simulink model "sb_cross_mult_core"  (R2012b)
settings: Solver=ode45  StartTime=0.0  StopTime=10.0  RelTol=1e-3
libraries: xbsIndex_r4 x485, casper_library_misc x72
(part 1 of 5)
settings Model: Creator=jack  LastModifiedBy=jack

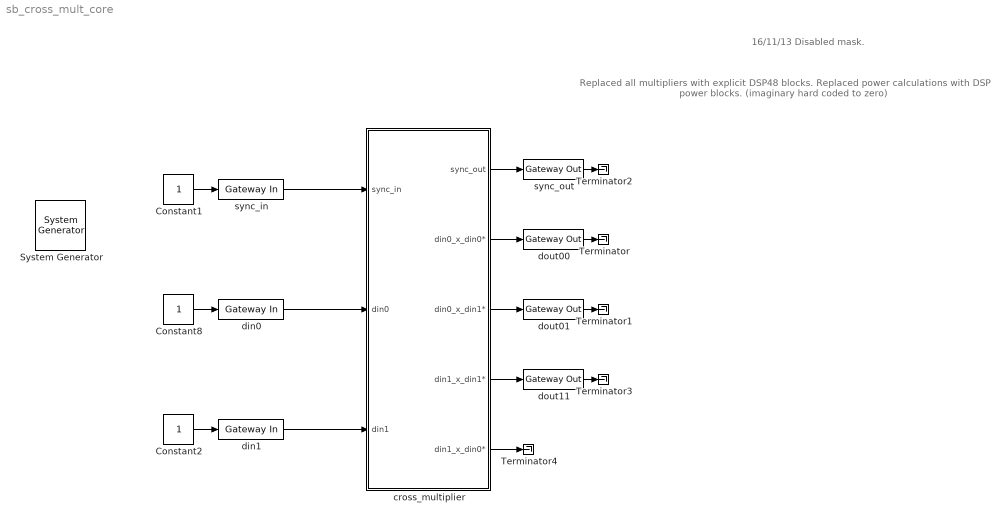
== system sb_cross_mult_core ==
  note: Replaced all multipliers with explicit DSP48 blocks.
      | Replaced power calculations with DSP power blocks. (imaginary hard coded to zero)
  note: 16/11/13
      | Disabled mask.
  " System Generator" : xbsIndex_r4/ System Generator  Tag=genX  xilinxfamily=virtex6  part=xc6vsx475t  speed=-1  package=ff1759  synthesis_tool=XST  clock_wrapper=Clock Enables  directory=./sb_cross_mult_core  proj_type=Project Navigator  Synth_file=XST Defaults  Impl_file=ISE Defaults  testbench=off  simulink_period=1  sysclk_period=3.2  dcm_input_clock_period=10  incr_netlist=off  trim_vbits=Everywhere in SubSystem  dbl_ovrd=According to Block Masks  core_generation=According to Block Masks  run_coregen=off  deprecated_control=off  eval_field=0  block_type=sysgen
  Constant1 : Constant
  Constant2 : Constant
  Constant8 : Constant
  Terminator{,1..4} (5 alike) : Terminator
  cross_multiplier : Subsystem  mask(cross_multiplier){streams=2, aggregation=8, bit_width_in=4, binary_point_in=3, bit_width_out=9, binary_point_out=6, mult_latency=3, add_latency=1, overflow=Wrap, quantisation=Truncate, conv_latency=0}
      mask prompts: streams "Number input streams"; aggregation "Aggregation per stream"; bit_width_in "Bit width in"; binary_point_in "Binary point in"; bit_width_out "Bit width out"; binary_point_out "Binary point out"; mult_latency "Multiplier latency"; add_latency "Adder latency"; overflow "Overflow behaviour"; quantisation "Quantisation behaviour"; conv_latency "Bit width conversion latency"
      mask help: Cross multiplies aggregated complex input streams.
      mask init:
      | % cross_multiplier_init(gcb, ...
      | %     'streams', streams, ...
      | %     'aggregation', aggregation, ...
      | %     'bit_width_in', bit_width_in, ...
      | %     'binary_point_in', binary_point_in, ...
      | %     'bit_width_out', bit_width_out, ...
      | %     'binary_point_out', binary_point_out, ...
      | %     'mult_latency', mult_latency, ...
      | %     'add_latency', add_latency, ...
      | %     'overflow', overflow, ...
      | %     'quantisation', quantisation, ...
      | %     'conv_latency', conv_latency);
      mask TypeOptions overflow: Wrap | Saturate | Error
      mask TypeOptions quantisation: Truncate | Round  (unbiased: +/- Inf) | Round  (unbiased: even values)
  din0 : xbsIndex_r4/Gateway In  gui_display_data_type=Fixed-point  arith_type=Unsigned  n_bits=8*8  bin_pt=0  preci_type=Single  exp_width=8  frac_width=24  quantization="Round  (unbiased: +/- Inf)"  overflow=Saturate  period=1  dbl_ovrd=off  timing_constraint=None  locs_specified=off  LOCs={}  UseAsADC=off  ADCChannel='1'  inherit_from_input=off  hdl_port=on  block_type=gatewayin
  din1 : xbsIndex_r4/Gateway In  gui_display_data_type=Fixed-point  arith_type=Unsigned  n_bits=8*8  bin_pt=0  preci_type=Single  exp_width=8  frac_width=24  quantization="Round  (unbiased: +/- Inf)"  overflow=Saturate  period=1  dbl_ovrd=off  timing_constraint=None  locs_specified=off  LOCs={}  UseAsADC=off  ADCChannel='1'  inherit_from_input=off  hdl_port=on  block_type=gatewayin
  dout00 : xbsIndex_r4/Gateway Out  inherit_from_input=off  hdl_port=on  timing_constraint=None  locs_specified=off  LOCs={}  UseAsDAC=off  DACChannel='1'  block_type=gatewayout
  dout01 : xbsIndex_r4/Gateway Out  inherit_from_input=off  hdl_port=on  timing_constraint=None  locs_specified=off  LOCs={}  UseAsDAC=off  DACChannel='1'  block_type=gatewayout
  dout11 : xbsIndex_r4/Gateway Out  inherit_from_input=off  hdl_port=on  timing_constraint=None  locs_specified=off  LOCs={}  UseAsDAC=off  DACChannel='1'  block_type=gatewayout
  sync_in : xbsIndex_r4/Gateway In  gui_display_data_type=Boolean  arith_type=Boolean  n_bits=16  bin_pt=14  preci_type=Single  exp_width=8  frac_width=24  quantization="Round  (unbiased: +/- Inf)"  overflow=Saturate  period=1  dbl_ovrd=off  timing_constraint=None  locs_specified=off  LOCs={}  UseAsADC=off  ADCChannel='1'  inherit_from_input=off  hdl_port=on  block_type=gatewayin
  sync_out : xbsIndex_r4/Gateway Out  inherit_from_input=off  hdl_port=on  timing_constraint=None  locs_specified=off  LOCs={}  UseAsDAC=off  DACChannel='1'  block_type=gatewayout
  wires:
  Constant1/1 -> sync_in/1
  dout00/1 -> Terminator/1
  sync_out/1 -> Terminator2/1
  Constant8/1 -> din0/1
  cross_multiplier/1(sync_out) -> sync_out/1
  cross_multiplier/2(din0_x_din0*) -> dout00/1
  dout01/1 -> Terminator1/1
  cross_multiplier/3(din0_x_din1*) -> dout01/1
  dout11/1 -> Terminator3/1
  cross_multiplier/4(din1_x_din1*) -> dout11/1
  cross_multiplier/5(din1_x_din0*) -> Terminator4/1
  sync_in/1 -> cross_multiplier/1(sync_in)
  din0/1 -> cross_multiplier/2(din0)
  Constant2/1 -> din1/1
  din1/1 -> cross_multiplier/3(din1)

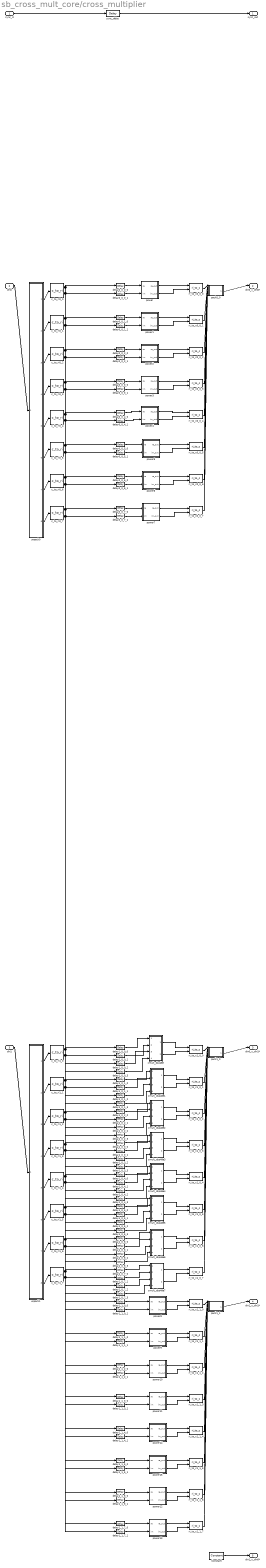
== system sb_cross_mult_core/cross_multiplier ==
  sync_in : Inport
  din0 : Inport  Port=2
  din1 : Inport  Port=3
  Constant : xbsIndex_r4/Constant  const=0  gui_display_data_type=Fixed-point  arith_type=Unsigned  n_bits=2*9*8  bin_pt=0  preci_type=Single  exp_width=8  frac_width=24  explicit_period=on  period=1  equ=P=C  opselect=C  inp2=PCIN>>17  opr=+  inp1=P  carry=CIN  dbl_ovrd=off  block_type=constant
  c_to_ri0_{0..7} (8 alike) : casper_library_misc/c_to_ri  n_bits=bit_width_in  bin_pt=binary_point_in
      settings: AttributesFormatString=4_3 r/i
  c_to_ri1_{0..7} (8 alike) : casper_library_misc/c_to_ri  n_bits=bit_width_in  bin_pt=binary_point_in
      settings: AttributesFormatString=4_3 r/i
  cmult_dsp48e : Subsystem  AncestorBlock=casper_library_multipliers/cmult_dsp48e  mask(cmult_dsp48e){n_bits_a=4, bin_pt_a=3, n_bits_b=4, bin_pt_b=3, conjugated=on, full_precision=on, n_bits_c=37, bin_pt_c=34, quantization=Truncate, overflow=Wrap, cast_latency=0}
      mask prompts: n_bits_a "Bit width 'a'"; bin_pt_a "Binary point 'a'"; n_bits_b "Bit width 'b'"; bin_pt_b "Binary point 'b'"; conjugated "Conjugate"; full_precision "Full precision"; n_bits_c "Bit width out"; bin_pt_c "Binary point out"; cast_latency "Cast Latency"
      mask help:
      | Multiplies two complex numbers using 4 DSP48Es.
      | Conjugation is optional.
      |
      | Re{a} and Im{a} can be up to 25 bits.
      | Re{b} and Im{b} can be up to 18 bits.
      mask init:
      | cmult_dsp48e_init(gcb, ...
      |     'n_bits_a', n_bits_a, ...
      |     'bin_pt_a', bin_pt_a, ...
      |     'n_bits_b', n_bits_b, ...
      |     'bin_pt_b', bin_pt_b, ...
      |     'conjugated', conjugated, ...
      |     'full_precision', full_precision, ...
      |     'n_bits_c', n_bits_c, ...
      |     'bin_pt_c', bin_pt_c, ...
      |     'quantization', quantization, ...
      |     'overflow', overflow, ...
      |     'cast_latency', cast_latency);
      settings: AttributesFormatString=|
      | 4_3 * 4_3 ==> 9_6
      | Latency=4
      mask Callback full_precision:
      | full_precision = get_param(gcb, 'full_precision');
      | 
      | if strcmp(full_precision, 'on'),
      |     not_full_precision = 'off';
      | else
      |     not_full_precision = 'on';
      | end
      | 
      | set_param_state(gcb, 'n_bits_c', not_full_precision);
      | set_param_state(gcb, 'bin_pt_c', not_full_precision);
      | set_param_state(gcb, 'quantization', not_full_precision);
      | set_param_state(gcb, 'overflow', not_full_precision);
      | set_param_state(gcb, 'cast_latency', not_full_precision);
      mask TypeOptions quantization: Truncate | Round  (unbiased: +/- Inf) | Round  (unbiased: Even Values)
      mask TypeOptions overflow: Wrap | Saturate | Flag as error
  cmult_dsp48e1 : Subsystem  AncestorBlock=casper_library_multipliers/cmult_dsp48e  mask(cmult_dsp48e){n_bits_a=4, bin_pt_a=3, n_bits_b=4, bin_pt_b=3, conjugated=on, full_precision=on, n_bits_c=37, bin_pt_c=34, quantization=Truncate, overflow=Wrap, cast_latency=0}
      mask prompts: n_bits_a "Bit width 'a'"; bin_pt_a "Binary point 'a'"; n_bits_b "Bit width 'b'"; bin_pt_b "Binary point 'b'"; conjugated "Conjugate"; full_precision "Full precision"; n_bits_c "Bit width out"; bin_pt_c "Binary point out"; cast_latency "Cast Latency"
      mask help:
      | Multiplies two complex numbers using 4 DSP48Es.
      | Conjugation is optional.
      |
      | Re{a} and Im{a} can be up to 25 bits.
      | Re{b} and Im{b} can be up to 18 bits.
      mask init: same as sb_cross_mult_core/cross_multiplier/cmult_dsp48e
      settings: AttributesFormatString=|
      | 4_3 * 4_3 ==> 9_6
      | Latency=4
      mask Callback full_precision:
      | full_precision = get_param(gcb, 'full_precision');
      | 
      | if strcmp(full_precision, 'on'),
      |     not_full_precision = 'off';
      | else
      |     not_full_precision = 'on';
      | end
      | 
      | set_param_state(gcb, 'n_bits_c', not_full_precision);
      | set_param_state(gcb, 'bin_pt_c', not_full_precision);
      | set_param_state(gcb, 'quantization', not_full_precision);
      | set_param_state(gcb, 'overflow', not_full_precision);
      | set_param_state(gcb, 'cast_latency', not_full_precision);
      mask TypeOptions quantization: Truncate | Round  (unbiased: +/- Inf) | Round  (unbiased: Even Values)
      mask TypeOptions overflow: Wrap | Saturate | Flag as error
  cmult_dsp48e2 : Subsystem  AncestorBlock=casper_library_multipliers/cmult_dsp48e  mask(cmult_dsp48e){n_bits_a=4, bin_pt_a=3, n_bits_b=4, bin_pt_b=3, conjugated=on, full_precision=on, n_bits_c=37, bin_pt_c=34, quantization=Truncate, overflow=Wrap, cast_latency=0}
      mask prompts: n_bits_a "Bit width 'a'"; bin_pt_a "Binary point 'a'"; n_bits_b "Bit width 'b'"; bin_pt_b "Binary point 'b'"; conjugated "Conjugate"; full_precision "Full precision"; n_bits_c "Bit width out"; bin_pt_c "Binary point out"; cast_latency "Cast Latency"
      mask help:
      | Multiplies two complex numbers using 4 DSP48Es.
      | Conjugation is optional.
      |
      | Re{a} and Im{a} can be up to 25 bits.
      | Re{b} and Im{b} can be up to 18 bits.
      mask init: same as sb_cross_mult_core/cross_multiplier/cmult_dsp48e
      settings: AttributesFormatString=|
      | 4_3 * 4_3 ==> 9_6
      | Latency=4
      mask Callback full_precision:
      | full_precision = get_param(gcb, 'full_precision');
      | 
      | if strcmp(full_precision, 'on'),
      |     not_full_precision = 'off';
      | else
      |     not_full_precision = 'on';
      | end
      | 
      | set_param_state(gcb, 'n_bits_c', not_full_precision);
      | set_param_state(gcb, 'bin_pt_c', not_full_precision);
      | set_param_state(gcb, 'quantization', not_full_precision);
      | set_param_state(gcb, 'overflow', not_full_precision);
      | set_param_state(gcb, 'cast_latency', not_full_precision);
      mask TypeOptions quantization: Truncate | Round  (unbiased: +/- Inf) | Round  (unbiased: Even Values)
      mask TypeOptions overflow: Wrap | Saturate | Flag as error
  cmult_dsp48e3 : Subsystem  AncestorBlock=casper_library_multipliers/cmult_dsp48e  mask(cmult_dsp48e){n_bits_a=4, bin_pt_a=3, n_bits_b=4, bin_pt_b=3, conjugated=on, full_precision=on, n_bits_c=37, bin_pt_c=34, quantization=Truncate, overflow=Wrap, cast_latency=0}
      mask prompts: n_bits_a "Bit width 'a'"; bin_pt_a "Binary point 'a'"; n_bits_b "Bit width 'b'"; bin_pt_b "Binary point 'b'"; conjugated "Conjugate"; full_precision "Full precision"; n_bits_c "Bit width out"; bin_pt_c "Binary point out"; cast_latency "Cast Latency"
      mask help:
      | Multiplies two complex numbers using 4 DSP48Es.
      | Conjugation is optional.
      |
      | Re{a} and Im{a} can be up to 25 bits.
      | Re{b} and Im{b} can be up to 18 bits.
      mask init: same as sb_cross_mult_core/cross_multiplier/cmult_dsp48e
      settings: AttributesFormatString=|
      | 4_3 * 4_3 ==> 9_6
      | Latency=4
      mask Callback full_precision:
      | full_precision = get_param(gcb, 'full_precision');
      | 
      | if strcmp(full_precision, 'on'),
      |     not_full_precision = 'off';
      | else
      |     not_full_precision = 'on';
      | end
      | 
      | set_param_state(gcb, 'n_bits_c', not_full_precision);
      | set_param_state(gcb, 'bin_pt_c', not_full_precision);
      | set_param_state(gcb, 'quantization', not_full_precision);
      | set_param_state(gcb, 'overflow', not_full_precision);
      | set_param_state(gcb, 'cast_latency', not_full_precision);
      mask TypeOptions quantization: Truncate | Round  (unbiased: +/- Inf) | Round  (unbiased: Even Values)
      mask TypeOptions overflow: Wrap | Saturate | Flag as error
  cmult_dsp48e4 : Subsystem  AncestorBlock=casper_library_multipliers/cmult_dsp48e  mask(cmult_dsp48e){n_bits_a=4, bin_pt_a=3, n_bits_b=4, bin_pt_b=3, conjugated=on, full_precision=on, n_bits_c=37, bin_pt_c=34, quantization=Truncate, overflow=Wrap, cast_latency=0}
      mask prompts: n_bits_a "Bit width 'a'"; bin_pt_a "Binary point 'a'"; n_bits_b "Bit width 'b'"; bin_pt_b "Binary point 'b'"; conjugated "Conjugate"; full_precision "Full precision"; n_bits_c "Bit width out"; bin_pt_c "Binary point out"; cast_latency "Cast Latency"
      mask help:
      | Multiplies two complex numbers using 4 DSP48Es.
      | Conjugation is optional.
      |
      | Re{a} and Im{a} can be up to 25 bits.
      | Re{b} and Im{b} can be up to 18 bits.
      mask init: same as sb_cross_mult_core/cross_multiplier/cmult_dsp48e
      settings: AttributesFormatString=|
      | 4_3 * 4_3 ==> 9_6
      | Latency=4
      mask Callback full_precision:
      | full_precision = get_param(gcb, 'full_precision');
      | 
      | if strcmp(full_precision, 'on'),
      |     not_full_precision = 'off';
      | else
      |     not_full_precision = 'on';
      | end
      | 
      | set_param_state(gcb, 'n_bits_c', not_full_precision);
      | set_param_state(gcb, 'bin_pt_c', not_full_precision);
      | set_param_state(gcb, 'quantization', not_full_precision);
      | set_param_state(gcb, 'overflow', not_full_precision);
      | set_param_state(gcb, 'cast_latency', not_full_precision);
      mask TypeOptions quantization: Truncate | Round  (unbiased: +/- Inf) | Round  (unbiased: Even Values)
      mask TypeOptions overflow: Wrap | Saturate | Flag as error
  cmult_dsp48e5 : Subsystem  AncestorBlock=casper_library_multipliers/cmult_dsp48e  mask(cmult_dsp48e){n_bits_a=4, bin_pt_a=3, n_bits_b=4, bin_pt_b=3, conjugated=on, full_precision=on, n_bits_c=37, bin_pt_c=34, quantization=Truncate, overflow=Wrap, cast_latency=0}
      mask prompts: n_bits_a "Bit width 'a'"; bin_pt_a "Binary point 'a'"; n_bits_b "Bit width 'b'"; bin_pt_b "Binary point 'b'"; conjugated "Conjugate"; full_precision "Full precision"; n_bits_c "Bit width out"; bin_pt_c "Binary point out"; cast_latency "Cast Latency"
      mask help:
      | Multiplies two complex numbers using 4 DSP48Es.
      | Conjugation is optional.
      |
      | Re{a} and Im{a} can be up to 25 bits.
      | Re{b} and Im{b} can be up to 18 bits.
      mask init: same as sb_cross_mult_core/cross_multiplier/cmult_dsp48e
      settings: AttributesFormatString=|
      | 4_3 * 4_3 ==> 9_6
      | Latency=4
      mask Callback full_precision:
      | full_precision = get_param(gcb, 'full_precision');
      | 
      | if strcmp(full_precision, 'on'),
      |     not_full_precision = 'off';
      | else
      |     not_full_precision = 'on';
      | end
      | 
      | set_param_state(gcb, 'n_bits_c', not_full_precision);
      | set_param_state(gcb, 'bin_pt_c', not_full_precision);
      | set_param_state(gcb, 'quantization', not_full_precision);
      | set_param_state(gcb, 'overflow', not_full_precision);
      | set_param_state(gcb, 'cast_latency', not_full_precision);
      mask TypeOptions quantization: Truncate | Round  (unbiased: +/- Inf) | Round  (unbiased: Even Values)
      mask TypeOptions overflow: Wrap | Saturate | Flag as error
  cmult_dsp48e6 : Subsystem  AncestorBlock=casper_library_multipliers/cmult_dsp48e  mask(cmult_dsp48e){n_bits_a=4, bin_pt_a=3, n_bits_b=4, bin_pt_b=3, conjugated=on, full_precision=on, n_bits_c=37, bin_pt_c=34, quantization=Truncate, overflow=Wrap, cast_latency=0}
      mask prompts: n_bits_a "Bit width 'a'"; bin_pt_a "Binary point 'a'"; n_bits_b "Bit width 'b'"; bin_pt_b "Binary point 'b'"; conjugated "Conjugate"; full_precision "Full precision"; n_bits_c "Bit width out"; bin_pt_c "Binary point out"; cast_latency "Cast Latency"
      mask help:
      | Multiplies two complex numbers using 4 DSP48Es.
      | Conjugation is optional.
      |
      | Re{a} and Im{a} can be up to 25 bits.
      | Re{b} and Im{b} can be up to 18 bits.
      mask init: same as sb_cross_mult_core/cross_multiplier/cmult_dsp48e
      settings: AttributesFormatString=|
      | 4_3 * 4_3 ==> 9_6
      | Latency=4
      mask Callback full_precision:
      | full_precision = get_param(gcb, 'full_precision');
      | 
      | if strcmp(full_precision, 'on'),
      |     not_full_precision = 'off';
      | else
      |     not_full_precision = 'on';
      | end
      | 
      | set_param_state(gcb, 'n_bits_c', not_full_precision);
      | set_param_state(gcb, 'bin_pt_c', not_full_precision);
      | set_param_state(gcb, 'quantization', not_full_precision);
      | set_param_state(gcb, 'overflow', not_full_precision);
      | set_param_state(gcb, 'cast_latency', not_full_precision);
      mask TypeOptions quantization: Truncate | Round  (unbiased: +/- Inf) | Round  (unbiased: Even Values)
      mask TypeOptions overflow: Wrap | Saturate | Flag as error
  cmult_dsp48e7 : Subsystem  AncestorBlock=casper_library_multipliers/cmult_dsp48e  mask(cmult_dsp48e){n_bits_a=4, bin_pt_a=3, n_bits_b=4, bin_pt_b=3, conjugated=on, full_precision=on, n_bits_c=37, bin_pt_c=34, quantization=Truncate, overflow=Wrap, cast_latency=0}
      mask prompts: n_bits_a "Bit width 'a'"; bin_pt_a "Binary point 'a'"; n_bits_b "Bit width 'b'"; bin_pt_b "Binary point 'b'"; conjugated "Conjugate"; full_precision "Full precision"; n_bits_c "Bit width out"; bin_pt_c "Binary point out"; cast_latency "Cast Latency"
      mask help:
      | Multiplies two complex numbers using 4 DSP48Es.
      | Conjugation is optional.
      |
      | Re{a} and Im{a} can be up to 25 bits.
      | Re{b} and Im{b} can be up to 18 bits.
      mask init: same as sb_cross_mult_core/cross_multiplier/cmult_dsp48e
      settings: AttributesFormatString=|
      | 4_3 * 4_3 ==> 9_6
      | Latency=4
      mask Callback full_precision:
      | full_precision = get_param(gcb, 'full_precision');
      | 
      | if strcmp(full_precision, 'on'),
      |     not_full_precision = 'off';
      | else
      |     not_full_precision = 'on';
      | end
      | 
      | set_param_state(gcb, 'n_bits_c', not_full_precision);
      | set_param_state(gcb, 'bin_pt_c', not_full_precision);
      | set_param_state(gcb, 'quantization', not_full_precision);
      | set_param_state(gcb, 'overflow', not_full_precision);
      | set_param_state(gcb, 'cast_latency', not_full_precision);
      mask TypeOptions quantization: Truncate | Round  (unbiased: +/- Inf) | Round  (unbiased: Even Values)
      mask TypeOptions overflow: Wrap | Saturate | Flag as error
  delay0_0_0_0 : xbsIndex_r4/Delay  rst=off  infoeditControl=Selection of Reset will increase slice count due to use of real FFs and instead of SRLs  en=off  latency=1  dbl_ovrd=off  reg_retiming=off  block_type=delay
  delay0_0_0_1 : xbsIndex_r4/Delay  rst=off  infoeditControl=Selection of Reset will increase slice count due to use of real FFs and instead of SRLs  en=off  latency=1  dbl_ovrd=off  reg_retiming=off  block_type=delay
  delay0_0_1_0 : xbsIndex_r4/Delay  rst=off  infoeditControl=Selection of Reset will increase slice count due to use of real FFs and instead of SRLs  en=off  latency=1  dbl_ovrd=off  reg_retiming=off  block_type=delay
  delay0_0_1_1 : xbsIndex_r4/Delay  rst=off  infoeditControl=Selection of Reset will increase slice count due to use of real FFs and instead of SRLs  en=off  latency=1  dbl_ovrd=off  reg_retiming=off  block_type=delay
  delay0_0_2_0 : xbsIndex_r4/Delay  rst=off  infoeditControl=Selection of Reset will increase slice count due to use of real FFs and instead of SRLs  en=off  latency=1  dbl_ovrd=off  reg_retiming=off  block_type=delay
  delay0_0_2_1 : xbsIndex_r4/Delay  rst=off  infoeditControl=Selection of Reset will increase slice count due to use of real FFs and instead of SRLs  en=off  latency=1  dbl_ovrd=off  reg_retiming=off  block_type=delay
  delay0_0_3_0 : xbsIndex_r4/Delay  rst=off  infoeditControl=Selection of Reset will increase slice count due to use of real FFs and instead of SRLs  en=off  latency=1  dbl_ovrd=off  reg_retiming=off  block_type=delay
  delay0_0_3_1 : xbsIndex_r4/Delay  rst=off  infoeditControl=Selection of Reset will increase slice count due to use of real FFs and instead of SRLs  en=off  latency=1  dbl_ovrd=off  reg_retiming=off  block_type=delay
  delay0_0_4_0 : xbsIndex_r4/Delay  rst=off  infoeditControl=Selection of Reset will increase slice count due to use of real FFs and instead of SRLs  en=off  latency=1  dbl_ovrd=off  reg_retiming=off  block_type=delay
  delay0_0_4_1 : xbsIndex_r4/Delay  rst=off  infoeditControl=Selection of Reset will increase slice count due to use of real FFs and instead of SRLs  en=off  latency=1  dbl_ovrd=off  reg_retiming=off  block_type=delay
  delay0_0_5_0 : xbsIndex_r4/Delay  rst=off  infoeditControl=Selection of Reset will increase slice count due to use of real FFs and instead of SRLs  en=off  latency=1  dbl_ovrd=off  reg_retiming=off  block_type=delay
  delay0_0_5_1 : xbsIndex_r4/Delay  rst=off  infoeditControl=Selection of Reset will increase slice count due to use of real FFs and instead of SRLs  en=off  latency=1  dbl_ovrd=off  reg_retiming=off  block_type=delay
  delay0_0_6_0 : xbsIndex_r4/Delay  rst=off  infoeditControl=Selection of Reset will increase slice count due to use of real FFs and instead of SRLs  en=off  latency=1  dbl_ovrd=off  reg_retiming=off  block_type=delay
  delay0_0_6_1 : xbsIndex_r4/Delay  rst=off  infoeditControl=Selection of Reset will increase slice count due to use of real FFs and instead of SRLs  en=off  latency=1  dbl_ovrd=off  reg_retiming=off  block_type=delay
  delay0_0_7_0 : xbsIndex_r4/Delay  rst=off  infoeditControl=Selection of Reset will increase slice count due to use of real FFs and instead of SRLs  en=off  latency=1  dbl_ovrd=off  reg_retiming=off  block_type=delay
  delay0_0_7_1 : xbsIndex_r4/Delay  rst=off  infoeditControl=Selection of Reset will increase slice count due to use of real FFs and instead of SRLs  en=off  latency=1  dbl_ovrd=off  reg_retiming=off  block_type=delay
  delay1_0_0_{0..3} (4 alike) : xbsIndex_r4/Delay  rst=off  infoeditControl=Selection of Reset will increase slice count due to use of real FFs and instead of SRLs  en=off  latency=1  dbl_ovrd=off  reg_retiming=off  block_type=delay
  delay1_0_1_{0..3} (4 alike) : xbsIndex_r4/Delay  rst=off  infoeditControl=Selection of Reset will increase slice count due to use of real FFs and instead of SRLs  en=off  latency=1  dbl_ovrd=off  reg_retiming=off  block_type=delay
  delay1_0_2_{0..3} (4 alike) : xbsIndex_r4/Delay  rst=off  infoeditControl=Selection of Reset will increase slice count due to use of real FFs and instead of SRLs  en=off  latency=1  dbl_ovrd=off  reg_retiming=off  block_type=delay
  delay1_0_3_{0..3} (4 alike) : xbsIndex_r4/Delay  rst=off  infoeditControl=Selection of Reset will increase slice count due to use of real FFs and instead of SRLs  en=off  latency=1  dbl_ovrd=off  reg_retiming=off  block_type=delay
  delay1_0_4_{0..3} (4 alike) : xbsIndex_r4/Delay  rst=off  infoeditControl=Selection of Reset will increase slice count due to use of real FFs and instead of SRLs  en=off  latency=1  dbl_ovrd=off  reg_retiming=off  block_type=delay
  delay1_0_5_{0..3} (4 alike) : xbsIndex_r4/Delay  rst=off  infoeditControl=Selection of Reset will increase slice count due to use of real FFs and instead of SRLs  en=off  latency=1  dbl_ovrd=off  reg_retiming=off  block_type=delay
  delay1_0_6_{0..3} (4 alike) : xbsIndex_r4/Delay  rst=off  infoeditControl=Selection of Reset will increase slice count due to use of real FFs and instead of SRLs  en=off  latency=1  dbl_ovrd=off  reg_retiming=off  block_type=delay
  delay1_0_7_{0..3} (4 alike) : xbsIndex_r4/Delay  rst=off  infoeditControl=Selection of Reset will increase slice count due to use of real FFs and instead of SRLs  en=off  latency=1  dbl_ovrd=off  reg_retiming=off  block_type=delay
  delay1_1_0_0 : xbsIndex_r4/Delay  rst=off  infoeditControl=Selection of Reset will increase slice count due to use of real FFs and instead of SRLs  en=off  latency=1  dbl_ovrd=off  reg_retiming=off  block_type=delay
  delay1_1_0_1 : xbsIndex_r4/Delay  rst=off  infoeditControl=Selection of Reset will increase slice count due to use of real FFs and instead of SRLs  en=off  latency=1  dbl_ovrd=off  reg_retiming=off  block_type=delay
  delay1_1_1_0 : xbsIndex_r4/Delay  rst=off  infoeditControl=Selection of Reset will increase slice count due to use of real FFs and instead of SRLs  en=off  latency=1  dbl_ovrd=off  reg_retiming=off  block_type=delay
  delay1_1_1_1 : xbsIndex_r4/Delay  rst=off  infoeditControl=Selection of Reset will increase slice count due to use of real FFs and instead of SRLs  en=off  latency=1  dbl_ovrd=off  reg_retiming=off  block_type=delay
  delay1_1_2_0 : xbsIndex_r4/Delay  rst=off  infoeditControl=Selection of Reset will increase slice count due to use of real FFs and instead of SRLs  en=off  latency=1  dbl_ovrd=off  reg_retiming=off  block_type=delay
  delay1_1_2_1 : xbsIndex_r4/Delay  rst=off  infoeditControl=Selection of Reset will increase slice count due to use of real FFs and instead of SRLs  en=off  latency=1  dbl_ovrd=off  reg_retiming=off  block_type=delay
  delay1_1_3_0 : xbsIndex_r4/Delay  rst=off  infoeditControl=Selection of Reset will increase slice count due to use of real FFs and instead of SRLs  en=off  latency=1  dbl_ovrd=off  reg_retiming=off  block_type=delay
  delay1_1_3_1 : xbsIndex_r4/Delay  rst=off  infoeditControl=Selection of Reset will increase slice count due to use of real FFs and instead of SRLs  en=off  latency=1  dbl_ovrd=off  reg_retiming=off  block_type=delay
  delay1_1_4_0 : xbsIndex_r4/Delay  rst=off  infoeditControl=Selection of Reset will increase slice count due to use of real FFs and instead of SRLs  en=off  latency=1  dbl_ovrd=off  reg_retiming=off  block_type=delay
  delay1_1_4_1 : xbsIndex_r4/Delay  rst=off  infoeditControl=Selection of Reset will increase slice count due to use of real FFs and instead of SRLs  en=off  latency=1  dbl_ovrd=off  reg_retiming=off  block_type=delay
  delay1_1_5_0 : xbsIndex_r4/Delay  rst=off  infoeditControl=Selection of Reset will increase slice count due to use of real FFs and instead of SRLs  en=off  latency=1  dbl_ovrd=off  reg_retiming=off  block_type=delay
  delay1_1_5_1 : xbsIndex_r4/Delay  rst=off  infoeditControl=Selection of Reset will increase slice count due to use of real FFs and instead of SRLs  en=off  latency=1  dbl_ovrd=off  reg_retiming=off  block_type=delay
  delay1_1_6_0 : xbsIndex_r4/Delay  rst=off  infoeditControl=Selection of Reset will increase slice count due to use of real FFs and instead of SRLs  en=off  latency=1  dbl_ovrd=off  reg_retiming=off  block_type=delay
  delay1_1_6_1 : xbsIndex_r4/Delay  rst=off  infoeditControl=Selection of Reset will increase slice count due to use of real FFs and instead of SRLs  en=off  latency=1  dbl_ovrd=off  reg_retiming=off  block_type=delay
  delay1_1_7_0 : xbsIndex_r4/Delay  rst=off  infoeditControl=Selection of Reset will increase slice count due to use of real FFs and instead of SRLs  en=off  latency=1  dbl_ovrd=off  reg_retiming=off  block_type=delay
  delay1_1_7_1 : xbsIndex_r4/Delay  rst=off  infoeditControl=Selection of Reset will increase slice count due to use of real FFs and instead of SRLs  en=off  latency=1  dbl_ovrd=off  reg_retiming=off  block_type=delay
  pack0_0 : Subsystem  AncestorBlock=casper_library_flow_control/bus_create  mask(bus_create){inputNum=aggregation}
      mask prompts: inputNum "Number of inputs:"
      mask init:
      | bus_create_init(gcb,...
      |     'inputNum', inputNum);
  pack1_0 : Subsystem  AncestorBlock=casper_library_flow_control/bus_create  mask(bus_create){inputNum=aggregation}
      mask prompts: inputNum "Number of inputs:"
      mask init:
      | bus_create_init(gcb,...
      |     'inputNum', inputNum);
  pack1_1 : Subsystem  AncestorBlock=casper_library_flow_control/bus_create  mask(bus_create){inputNum=aggregation}
      mask prompts: inputNum "Number of inputs:"
      mask init:
      | bus_create_init(gcb,...
      |     'inputNum', inputNum);
  power : Subsystem
  power1 : Subsystem
  power10 : Subsystem
  power11 : Subsystem
  power12 : Subsystem
  power13 : Subsystem
  power14 : Subsystem
  power15 : Subsystem
  power2 : Subsystem
  power3 : Subsystem
  power4 : Subsystem
  power5 : Subsystem
  power6 : Subsystem
  power7 : Subsystem
  power8 : Subsystem
  power9 : Subsystem
  ri_to_c0_0_{0..7} (8 alike) : casper_library_misc/ri_to_c
  ri_to_c1_0_{0..7} (8 alike) : casper_library_misc/ri_to_c
  ri_to_c1_1_{0..7} (8 alike) : casper_library_misc/ri_to_c
  sync_delay : xbsIndex_r4/Delay  rst=off  infoeditControl=Selection of Reset will increase slice count due to use of real FFs and instead of SRLs  en=off  latency=mult_latency+add_latency+1+conv_latency  dbl_ovrd=off  reg_retiming=off  block_type=delay
  unpack0 : Subsystem  AncestorBlock=casper_library_flow_control/bus_expand  mask(bus_expand){mode=divisions of equal size, outputNum=aggregation, outputWidth=bit_width_in*2, outputBinaryPt=0, outputArithmeticType=0, show_format=off, outputToWorkspace=off, variablePrefix=out, outputToModelAsWell=on}
      mask prompts: outputNum "Number of outputs:"; outputWidth "Output width:"; outputBinaryPt "Output binary point position:"; outputArithmeticType "Output arithmetic type (ufix=0, fix=1, bool=2):"; show_format "Print format string?"; outputToWorkspace "Output to workspace?"; variablePrefix "Variable name prefix:"; outputToModelAsWell "Output to model as well?"
      mask help:
      | Expands a 'bus' made using a bus_create or Xilinx
      | concat block.
      | The input will be divided into the specified number
      | of outputs with the specified arithmetic types.
      | Divisions are made from most significant bit.
      mask init:
      | bus_expand_init(gcb,...
      |     'mode', mode, ...
      |     'outputNum', outputNum, ...
      |     'outputWidth', outputWidth, ...
      |     'outputBinaryPt', outputBinaryPt, ...
      |     'outputArithmeticType', outputArithmeticType, ...
      |     'show_format', show_format, ...
      |     'outputToWorkspace', outputToWorkspace, ...
      |     'variablePrefix', variablePrefix, ...
      |     'outputToModelAsWell', outputToModelAsWell);
      settings: AttributesFormatString=8 outputs
      mask TypeOptions mode: divisions of equal size | divisions of arbitrary size
      mask Callback mode: bus_expand_callback();
      mask Callback outputWidth: bus_expand_callback();
      mask Callback outputToWorkspace: bus_expand_callback();
  unpack1 : Subsystem  AncestorBlock=casper_library_flow_control/bus_expand  mask(bus_expand){mode=divisions of equal size, outputNum=aggregation, outputWidth=bit_width_in*2, outputBinaryPt=0, outputArithmeticType=0, show_format=off, outputToWorkspace=off, variablePrefix=out, outputToModelAsWell=on}
      mask prompts: outputNum "Number of outputs:"; outputWidth "Output width:"; outputBinaryPt "Output binary point position:"; outputArithmeticType "Output arithmetic type (ufix=0, fix=1, bool=2):"; show_format "Print format string?"; outputToWorkspace "Output to workspace?"; variablePrefix "Variable name prefix:"; outputToModelAsWell "Output to model as well?"
      mask help:
      | Expands a 'bus' made using a bus_create or Xilinx
      | concat block.
      | The input will be divided into the specified number
      | of outputs with the specified arithmetic types.
      | Divisions are made from most significant bit.
      mask init: same as sb_cross_mult_core/cross_multiplier/unpack0
      settings: AttributesFormatString=8 outputs
      mask TypeOptions mode: divisions of equal size | divisions of arbitrary size
      mask Callback mode: bus_expand_callback();
      mask Callback outputWidth: bus_expand_callback();
      mask Callback outputToWorkspace: bus_expand_callback();
  sync_out : Outport
  din0_x_din0* : Outport  Port=2
  din0_x_din1* : Outport  Port=3
  din1_x_din1* : Outport  Port=4
  din1_x_din0* : Outport  Port=5
  wires:
  sync_in/1 -> sync_delay/1
  sync_delay/1 -> sync_out/1
  din0/1 -> unpack0/1(bus_in)
  unpack0/1(msb_out8) -> c_to_ri0_0/1
  unpack0/2(out7) -> c_to_ri0_1/1
  unpack0/3(out6) -> c_to_ri0_2/1
  unpack0/4(out5) -> c_to_ri0_3/1
  unpack0/5(out4) -> c_to_ri0_4/1
  unpack0/6(out3) -> c_to_ri0_5/1
  unpack0/7(out2) -> c_to_ri0_6/1
  unpack0/8(lsb_out1) -> c_to_ri0_7/1
  c_to_ri0_0/1 -> delay0_0_0_0/1, delay1_0_0_0/1
  c_to_ri0_0/2 -> delay0_0_0_1/1, delay1_0_0_1/1
  ri_to_c0_0_0/1 -> pack0_0/1(in1)
  c_to_ri0_1/1 -> delay0_0_1_0/1, delay1_0_1_0/1
  c_to_ri0_1/2 -> delay0_0_1_1/1, delay1_0_1_1/1
  ri_to_c0_0_1/1 -> pack0_0/2(in2)
  c_to_ri0_2/1 -> delay0_0_2_0/1, delay1_0_2_0/1
  c_to_ri0_2/2 -> delay0_0_2_1/1, delay1_0_2_1/1
  ri_to_c0_0_2/1 -> pack0_0/3(in3)
  c_to_ri0_3/1 -> delay0_0_3_0/1, delay1_0_3_0/1
  c_to_ri0_3/2 -> delay0_0_3_1/1, delay1_0_3_1/1
  ri_to_c0_0_3/1 -> pack0_0/4(in4)
  c_to_ri0_4/1 -> delay0_0_4_0/1, delay1_0_4_0/1
  c_to_ri0_4/2 -> delay0_0_4_1/1, delay1_0_4_1/1
  ri_to_c0_0_4/1 -> pack0_0/5(in5)
  c_to_ri0_5/1 -> delay0_0_5_0/1, delay1_0_5_0/1
  c_to_ri0_5/2 -> delay0_0_5_1/1, delay1_0_5_1/1
  ri_to_c0_0_5/1 -> pack0_0/6(in6)
  c_to_ri0_6/1 -> delay0_0_6_0/1, delay1_0_6_0/1
  c_to_ri0_6/2 -> delay0_0_6_1/1, delay1_0_6_1/1
  ri_to_c0_0_6/1 -> pack0_0/7(in7)
  c_to_ri0_7/1 -> delay0_0_7_0/1, delay1_0_7_0/1
  c_to_ri0_7/2 -> delay0_0_7_1/1, delay1_0_7_1/1
  ri_to_c0_0_7/1 -> pack0_0/8(in8)
  pack0_0/1(bus_out) -> din0_x_din0*/1
  din1/1 -> unpack1/1(bus_in)
  unpack1/1(msb_out8) -> c_to_ri1_0/1
  unpack1/2(out7) -> c_to_ri1_1/1
  unpack1/3(out6) -> c_to_ri1_2/1
  unpack1/4(out5) -> c_to_ri1_3/1
  unpack1/5(out4) -> c_to_ri1_4/1
  unpack1/6(out3) -> c_to_ri1_5/1
  unpack1/7(out2) -> c_to_ri1_6/1
  unpack1/8(lsb_out1) -> c_to_ri1_7/1
  c_to_ri1_0/1 -> delay1_0_0_2/1, delay1_1_0_0/1
  c_to_ri1_0/2 -> delay1_0_0_3/1, delay1_1_0_1/1
  ri_to_c1_0_0/1 -> pack1_0/1(in1)
  c_to_ri1_1/1 -> delay1_0_1_2/1, delay1_1_1_0/1
  c_to_ri1_1/2 -> delay1_0_1_3/1, delay1_1_1_1/1
  ri_to_c1_0_1/1 -> pack1_0/2(in2)
  c_to_ri1_2/1 -> delay1_0_2_2/1, delay1_1_2_0/1
  c_to_ri1_2/2 -> delay1_0_2_3/1, delay1_1_2_1/1
  ri_to_c1_0_2/1 -> pack1_0/3(in3)
  c_to_ri1_3/1 -> delay1_0_3_2/1, delay1_1_3_0/1
  c_to_ri1_3/2 -> delay1_0_3_3/1, delay1_1_3_1/1
  ri_to_c1_0_3/1 -> pack1_0/4(in4)
  c_to_ri1_4/1 -> delay1_0_4_2/1, delay1_1_4_0/1
  c_to_ri1_4/2 -> delay1_0_4_3/1, delay1_1_4_1/1
  ri_to_c1_0_4/1 -> pack1_0/5(in5)
  c_to_ri1_5/1 -> delay1_0_5_2/1, delay1_1_5_0/1
  c_to_ri1_5/2 -> delay1_0_5_3/1, delay1_1_5_1/1
  ri_to_c1_0_5/1 -> pack1_0/6(in6)
  c_to_ri1_6/1 -> delay1_0_6_2/1, delay1_1_6_0/1
  c_to_ri1_6/2 -> delay1_0_6_3/1, delay1_1_6_1/1
  ri_to_c1_0_6/1 -> pack1_0/7(in7)
  c_to_ri1_7/1 -> delay1_0_7_2/1, delay1_1_7_0/1
  c_to_ri1_7/2 -> delay1_0_7_3/1, delay1_1_7_1/1
  ri_to_c1_0_7/1 -> pack1_0/8(in8)
  pack1_0/1(bus_out) -> din0_x_din1*/1
  ri_to_c1_1_0/1 -> pack1_1/1(in1)
  ri_to_c1_1_1/1 -> pack1_1/2(in2)
  ri_to_c1_1_2/1 -> pack1_1/3(in3)
  ri_to_c1_1_3/1 -> pack1_1/4(in4)
  ri_to_c1_1_4/1 -> pack1_1/5(in5)
  ri_to_c1_1_5/1 -> pack1_1/6(in6)
  ri_to_c1_1_6/1 -> pack1_1/7(in7)
  ri_to_c1_1_7/1 -> pack1_1/8(in8)
  pack1_1/1(bus_out) -> din1_x_din1*/1
  delay0_0_0_0/1 -> power/1(re)
  delay0_0_0_1/1 -> power/2(im)
  power/1(re_out) -> ri_to_c0_0_0/1
  power/2(im_out) -> ri_to_c0_0_0/2
  delay0_0_1_1/1 -> power1/2(im)
  delay0_0_1_0/1 -> power1/1(re)
  power1/1(re_out) -> ri_to_c0_0_1/1
  power1/2(im_out) -> ri_to_c0_0_1/2
  delay0_0_2_0/1 -> power2/1(re)
  delay0_0_2_1/1 -> power2/2(im)
  power2/1(re_out) -> ri_to_c0_0_2/1
  power2/2(im_out) -> ri_to_c0_0_2/2
  delay0_0_3_0/1 -> power3/1(re)
  delay0_0_3_1/1 -> power3/2(im)
  power3/1(re_out) -> ri_to_c0_0_3/1
  power3/2(im_out) -> ri_to_c0_0_3/2
  delay0_0_4_0/1 -> power4/1(re)
  delay0_0_4_1/1 -> power4/2(im)
  power4/1(re_out) -> ri_to_c0_0_4/1
  power4/2(im_out) -> ri_to_c0_0_4/2
  delay0_0_5_0/1 -> power5/1(re)
  delay0_0_5_1/1 -> power5/2(im)
  power5/1(re_out) -> ri_to_c0_0_5/1
  power5/2(im_out) -> ri_to_c0_0_5/2
  delay0_0_6_0/1 -> power6/1(re)
  delay0_0_6_1/1 -> power6/2(im)
  power6/1(re_out) -> ri_to_c0_0_6/1
  power6/2(im_out) -> ri_to_c0_0_6/2
  power7/1(re_out) -> ri_to_c0_0_7/1
  power7/2(im_out) -> ri_to_c0_0_7/2
  delay0_0_7_1/1 -> power7/2(im)
  delay0_0_7_0/1 -> power7/1(re)
  delay1_0_0_0/1 -> cmult_dsp48e/1(a_re)
  delay1_0_0_1/1 -> cmult_dsp48e/2(a_im)
  delay1_0_0_2/1 -> cmult_dsp48e/3(b_re)
  delay1_0_0_3/1 -> cmult_dsp48e/4(b_im)
  cmult_dsp48e/2(c_im) -> ri_to_c1_0_0/2
  cmult_dsp48e/1(c_re) -> ri_to_c1_0_0/1
  delay1_0_1_0/1 -> cmult_dsp48e1/1(a_re)
  delay1_0_1_1/1 -> cmult_dsp48e1/2(a_im)
  delay1_0_1_2/1 -> cmult_dsp48e1/3(b_re)
  delay1_0_1_3/1 -> cmult_dsp48e1/4(b_im)
  cmult_dsp48e1/1(c_re) -> ri_to_c1_0_1/1
  cmult_dsp48e1/2(c_im) -> ri_to_c1_0_1/2
  delay1_0_2_0/1 -> cmult_dsp48e2/1(a_re)
  delay1_0_2_1/1 -> cmult_dsp48e2/2(a_im)
  delay1_0_2_2/1 -> cmult_dsp48e2/3(b_re)
  delay1_0_2_3/1 -> cmult_dsp48e2/4(b_im)
  cmult_dsp48e2/1(c_re) -> ri_to_c1_0_2/1
  cmult_dsp48e2/2(c_im) -> ri_to_c1_0_2/2
  delay1_0_3_0/1 -> cmult_dsp48e3/1(a_re)
  delay1_0_3_1/1 -> cmult_dsp48e3/2(a_im)
  delay1_0_3_2/1 -> cmult_dsp48e3/3(b_re)
  delay1_0_3_3/1 -> cmult_dsp48e3/4(b_im)
  cmult_dsp48e3/1(c_re) -> ri_to_c1_0_3/1
  cmult_dsp48e3/2(c_im) -> ri_to_c1_0_3/2
  delay1_0_4_0/1 -> cmult_dsp48e4/1(a_re)
  delay1_0_4_1/1 -> cmult_dsp48e4/2(a_im)
  delay1_0_4_2/1 -> cmult_dsp48e4/3(b_re)
  delay1_0_4_3/1 -> cmult_dsp48e4/4(b_im)
  cmult_dsp48e4/1(c_re) -> ri_to_c1_0_4/1
  cmult_dsp48e4/2(c_im) -> ri_to_c1_0_4/2
  delay1_0_5_0/1 -> cmult_dsp48e5/1(a_re)
  delay1_0_5_1/1 -> cmult_dsp48e5/2(a_im)
  delay1_0_5_2/1 -> cmult_dsp48e5/3(b_re)
  delay1_0_5_3/1 -> cmult_dsp48e5/4(b_im)
  cmult_dsp48e5/1(c_re) -> ri_to_c1_0_5/1
  cmult_dsp48e5/2(c_im) -> ri_to_c1_0_5/2
  delay1_0_6_0/1 -> cmult_dsp48e6/1(a_re)
  delay1_0_6_1/1 -> cmult_dsp48e6/2(a_im)
  delay1_0_6_2/1 -> cmult_dsp48e6/3(b_re)
  delay1_0_6_3/1 -> cmult_dsp48e6/4(b_im)
  cmult_dsp48e6/1(c_re) -> ri_to_c1_0_6/1
  cmult_dsp48e6/2(c_im) -> ri_to_c1_0_6/2
  delay1_0_7_0/1 -> cmult_dsp48e7/1(a_re)
  delay1_0_7_1/1 -> cmult_dsp48e7/2(a_im)
  delay1_0_7_2/1 -> cmult_dsp48e7/3(b_re)
  delay1_0_7_3/1 -> cmult_dsp48e7/4(b_im)
  cmult_dsp48e7/1(c_re) -> ri_to_c1_0_7/1
  cmult_dsp48e7/2(c_im) -> ri_to_c1_0_7/2
  delay1_1_0_0/1 -> power8/1(re)
  delay1_1_0_1/1 -> power8/2(im)
  power8/1(re_out) -> ri_to_c1_1_0/1
  power8/2(im_out) -> ri_to_c1_1_0/2
  delay1_1_1_0/1 -> power9/1(re)
  delay1_1_1_1/1 -> power9/2(im)
  power9/1(re_out) -> ri_to_c1_1_1/1
  power9/2(im_out) -> ri_to_c1_1_1/2
  delay1_1_2_0/1 -> power10/1(re)
  delay1_1_2_1/1 -> power10/2(im)
  power10/1(re_out) -> ri_to_c1_1_2/1
  power10/2(im_out) -> ri_to_c1_1_2/2
  delay1_1_3_0/1 -> power11/1(re)
  delay1_1_3_1/1 -> power11/2(im)
  power11/1(re_out) -> ri_to_c1_1_3/1
  power11/2(im_out) -> ri_to_c1_1_3/2
  delay1_1_4_0/1 -> power14/1(re)
  delay1_1_4_1/1 -> power14/2(im)
  power14/1(re_out) -> ri_to_c1_1_4/1
  power14/2(im_out) -> ri_to_c1_1_4/2
  delay1_1_5_0/1 -> power15/1(re)
  delay1_1_5_1/1 -> power15/2(im)
  power15/1(re_out) -> ri_to_c1_1_5/1
  power15/2(im_out) -> ri_to_c1_1_5/2
  delay1_1_6_1/1 -> power12/2(im)
  delay1_1_6_0/1 -> power12/1(re)
  power12/1(re_out) -> ri_to_c1_1_6/1
  power12/2(im_out) -> ri_to_c1_1_6/2
  delay1_1_7_0/1 -> power13/1(re)
  delay1_1_7_1/1 -> power13/2(im)
  power13/1(re_out) -> ri_to_c1_1_7/1
  power13/2(im_out) -> ri_to_c1_1_7/2
  Constant/1 -> din1_x_din0*/1
